simulink model "ADC_DAC"  (Simulink 7.4)
settings: Solver=ode1  SolverMode=SingleTasking  StartTime=0.0  StopTime=inf  FixedStep=0.01  MaxStep=0.02  RelTol=1e-3  AbsTol=1e-6
libraries: mc9s12tool x1
CloseFcn:
  | rtwprivate ssgencode ModelCloseRequest MC_AD
settings Model: Creator=Admin  LastModifiedBy=fw  SimulationMode=external
settings ConfigSet: Description=rtmc9s12target_R2009b
settings DataIOCC: LimitDataPoints=off  SaveOutput=off  SaveTime=off  SignalLoggingName=sigsOut
settings OptimizationCC: BlockReduction=off  BooleanDataType=off  InitFltsAndDblsToZero=on  OptimizeModelRefInitCode=on  LifeSpan=1
settings DebuggingCC: SaveWithParameterizedLinksMsg=none  SignalResolutionControl=TryResolveAllWithWarning  SolverPrmCheckMsg=none  MultiTaskDSMMsg=warning  MultiTaskCondExecSysMsg=none  StrictBusMsg=None
settings HardwareCC: ProdBitPerInt=16  ProdEndianess=BigEndian  ProdWordSize=16  ProdHWDeviceType=Motorola HC12
settings RTWCC: SystemTargetFile=mc9s12.tlc  GenerateMakefile=off  TemplateMakefile=mc9s12.tmf  ProcessScript=mc9s12_make_rtw_hook  IncludeERTFirstTime=on
settings CodeAppCC: IgnoreCustomStorageClasses=off
settings STFCustomTargetCC: TargetFcnLib=ansi_tfl_tmw.mat  ModelReferenceCompliant=off  IncludeMdlTerminateFcn=off  ERTCustomFileBanners=on  SupportNonInlinedSFcns=off  CPPClassGenCompliant=on  SystemTargetFile=mc9s12.tlc
settings ERTTargetCC: TargetFcnLib=ansi_tfl_tmw.mat  MultiwordLength=2048  ModelReferenceCompliant=off  ParMdlRefBuildCompliant=off  CompOptLevelCompliant=off  IncludeMdlTerminateFcn=off  CombineOutputUpdateFcns=off  ERTFirstTimeCompliant=off  SupportContinuousTime=on  ModelStepFunctionPrototypeControlCompliant=off  ExtMode=on  ExtModeMexFile=ext_serial_mc9s12_comm  ExtModeMexArgs=1,2,115200  InlinedParameterPlacement=NonHierarchical  ERTCustomFileTemplate=mc9s12_file_process.tlc  GRTInterface=on  ConvertIfToSwitch=off
settings CustomProperty: DataType=RTWOptions_EnumType_C__Users_fw__SVN_rtmc9s12-target_trunk_rtmc9s12_CW_R2009b_bin_mc9s12_1mc9s12_TargetBoard  Value=Dragon12Plus
settings EnumStrPairs: String=Dragon12

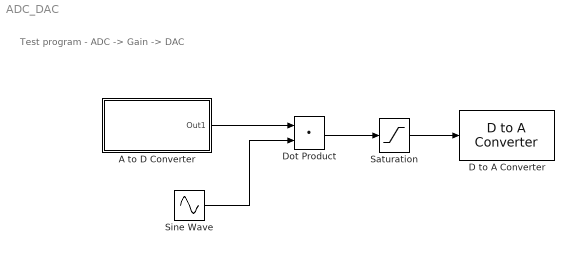
== system ADC_DAC ==
  note: Test program - ADC -> Gain -> DAC
  A to D Converter : Subsystem  Tag=mcTarget_adc  mask{bank=1, channels=2, use10bits=10 bits, normalize=max. output:  5, sampletime=0.01}
      mask prompts: bank "ADC bank"; channels "Channels ( 0 - 7 )"; use10bits "ADC resolution"; normalize "Normalization"; sampletime "Sample time"
      mask init:
      | [channelsStr, firstChannel, numChannels] = mbc_adcinput(channels);
      mask Help: web('adc_sfcn_9S12.html');
      mask StyleString: popup(0|1),edit,popup(10 bits|8 bits),popup(raw values|max. output:  1|max. output:  5),edit
      mask Display: disp(['A to D Converter\n' channelsStr])
  D to A Converter : mc9s12tool/D to A Converter  Tag=mcTarget_dac  SystemSampleTime=-1  sampletime=0.01  dac_channel=0  Vsat=5
  Dot Product : DotProduct  OutDataType=sfix(16)  OutScaling=2^-10  InputSameDT=on  OutDataTypeStr=Inherit: Inherit via internal rule
  Saturation : Saturate  UpperLimit=5  LowerLimit=0
  Sine Wave : Sin  Amplitude=1  Bias=0.5  Frequency=31.4  Phase=0  Samples=10  SampleTime=0  Offset=0
  wires:
  A to D Converter/1(Out1) -> Dot Product/1
  Dot Product/1 -> Saturation/1
  Saturation/1 -> D to A Converter/1
  Sine Wave/1 -> Dot Product/2

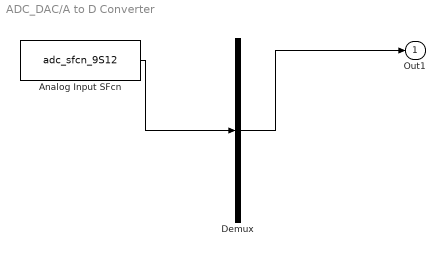
== system ADC_DAC/A to D Converter ==
  Analog Input SFcn : S-Function  Tag=mcTarget_adc  FunctionName=adc_sfcn_9S12  Parameters=bank-1, firstChannel, numChannels, use10bits-1, normalize, sampletime  EnableBusSupport=off
  Demux : Demux  Outputs=1
  Out1 : Outport  OutDataType=sfix(16)  OutScaling=2^0
  wires:
  Analog Input SFcn/1 -> Demux/1
  Demux/1 -> Out1/1
